simulink model "SbWModel"  (R2018a)
settings: Solver=FixedStepDiscrete  StartTime=0.0  StopTime=inf  FixedStep=0.002  RelTol=1e-3  EnableMultiTasking=on
values from neighbouring files (symbols this model uses):
  Bsc = 0.136    [SBWData.m]
  Im1 = 0.0021    [SBWData.m]
  Isw = 0.0079    [SBWData.m]
  Kb1 = 0.35    [SBWData.m]
  Ks1 = 3500    [SBWData.m]
  m = 1573    [STData.m]
  R1 = 4.6    [SBWData.m]
  RR = m*Csf    (= 34.606)    [STData.m]
  Tsmall = 0.001    [STData.m]
undefined symbols (not defined in the file or in its folder): Bm1, kt1, Tfr_c
settings Model: ExtModeTrigDuration=10000  Creator=srivats  LastModifiedBy=srivats
settings SolverCC: PositivePriorityOrder=on
settings RTWCC: SystemTargetFile=quarc_win64.tlc  TemplateMakefile=quarc_default_tmf  Description=QUARC Win64 Target
settings STFCustomTargetCC: TargetPreCompLibLocation=C:\PROGRA~3\QUARC\lib\2018a\win64\release  TargetLangStandard=C99 (ISO)  ConcurrentExecutionCompliant=on  SystemTargetFile=quarc_win64.tlc
settings GRTTargetCC: TargetPreCompLibLocation=C:\PROGRA~3\QUARC\lib\2018a\win64\release  ParMdlRefBuildCompliant=off  CompOptLevelCompliant=off  CombineOutputUpdateFcns=off  MatFileLogging=off  CPPClassGenCompliant=off  GRTInterface=on  UseToolchainInfoCompliant=off  ExtMode=on  ExtModeMexFile=quarc_comm

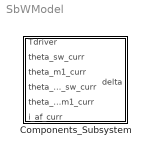
== system SbWModel ==
  Components_Subsystem : Subsystem

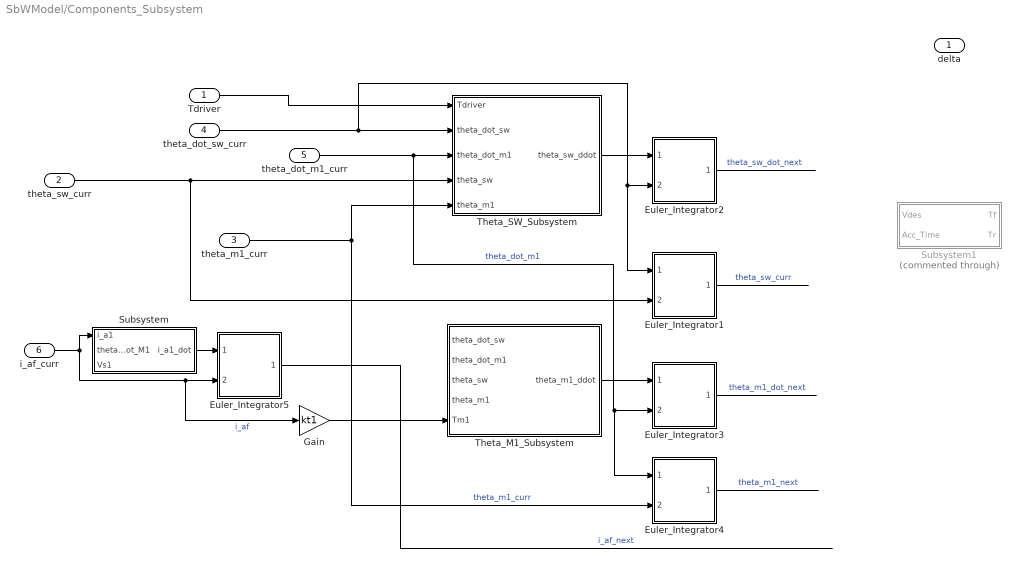
== system SbWModel/Components_Subsystem ==
  Tdriver : Inport
  theta_sw_curr : Inport  Port=2
  theta_m1_curr : Inport  Port=3
  theta_dot_sw_curr : Inport  Port=4
  theta_dot_m1_curr : Inport  Port=5
  i_af_curr : Inport  Port=6
  Euler_Integrator1 : Subsystem
  Euler_Integrator2 : Subsystem
  Euler_Integrator3 : Subsystem
  Euler_Integrator4 : Subsystem
  Euler_Integrator5 : Subsystem
  Gain : Gain  Gain=kt1
  Subsystem : Subsystem
  Subsystem1 : Subsystem  Commented=through
  Theta_M1_Subsystem : Subsystem
  Theta_SW_Subsystem : Subsystem
  delta : Outport
  wires:
  Tdriver/1 -> Theta_SW_Subsystem/1(Tdriver)
  theta_dot_sw_curr/1 -> Euler_Integrator1/1(state_dot), Euler_Integrator2/2(state_curr), Theta_SW_Subsystem/2(theta_dot_sw)
  theta_dot_m1_curr/1 -> Euler_Integrator4/1(state_dot), Euler_Integrator3/2(state_curr), Theta_SW_Subsystem/3(theta_dot_m1)  "theta_dot_m1"
  theta_sw_curr/1 -> Euler_Integrator1/2(state_curr), Theta_SW_Subsystem/4(theta_sw)
  theta_m1_curr/1 -> Euler_Integrator4/2(state_curr), Theta_SW_Subsystem/5(theta_m1)  "theta_m1_curr"
  Theta_SW_Subsystem/1(theta_sw_ddot) -> Euler_Integrator2/1(state_dot)
  Euler_Integrator2/1(state_next) -> ?  "theta_sw_dot_next"
  Euler_Integrator1/1(state_next) -> ?  "theta_sw_curr"
  Theta_M1_Subsystem/1("theta_m1_ddot ") -> Euler_Integrator3/1(state_dot)
  Euler_Integrator3/1(state_next) -> ?  "theta_m1_dot_next"
  Euler_Integrator4/1(state_next) -> ?  "theta_m1_next"
  i_af_curr/1 -> Gain/1, Euler_Integrator5/2(state_curr), Subsystem/1(i_a1)  "i_af"
  Subsystem/1(i_a1_dot) -> Euler_Integrator5/1(state_dot)
  Euler_Integrator5/1(state_next) -> ?  "i_af_next"
  Gain/1 -> Theta_M1_Subsystem/5(Tm1)

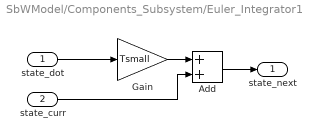
== system SbWModel/Components_Subsystem/Euler_Integrator1 ==
  state_dot : Inport
  state_curr : Inport  Port=2
  Add : Sum
  Gain : Gain  Gain=Tsmall
  state_next : Outport
  wires:
  state_dot/1 -> Gain/1
  Gain/1 -> Add/1
  state_curr/1 -> Add/2
  Add/1 -> state_next/1

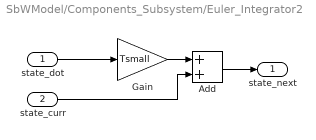
== system SbWModel/Components_Subsystem/Euler_Integrator2 ==
  state_dot : Inport
  state_curr : Inport  Port=2
  Add : Sum
  Gain : Gain  Gain=Tsmall
  state_next : Outport
  wires:
  state_dot/1 -> Gain/1
  Gain/1 -> Add/1
  state_curr/1 -> Add/2
  Add/1 -> state_next/1

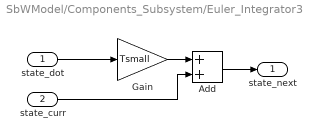
== system SbWModel/Components_Subsystem/Euler_Integrator3 ==
  state_dot : Inport
  state_curr : Inport  Port=2
  Add : Sum
  Gain : Gain  Gain=Tsmall
  state_next : Outport
  wires:
  state_dot/1 -> Gain/1
  Gain/1 -> Add/1
  state_curr/1 -> Add/2
  Add/1 -> state_next/1

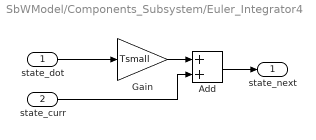
== system SbWModel/Components_Subsystem/Euler_Integrator4 ==
  state_dot : Inport
  state_curr : Inport  Port=2
  Add : Sum
  Gain : Gain  Gain=Tsmall
  state_next : Outport
  wires:
  state_dot/1 -> Gain/1
  Gain/1 -> Add/1
  state_curr/1 -> Add/2
  Add/1 -> state_next/1

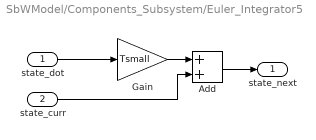
== system SbWModel/Components_Subsystem/Euler_Integrator5 ==
  state_dot : Inport
  state_curr : Inport  Port=2
  Add : Sum
  Gain : Gain  Gain=Tsmall
  state_next : Outport
  wires:
  state_dot/1 -> Gain/1
  Gain/1 -> Add/1
  state_curr/1 -> Add/2
  Add/1 -> state_next/1

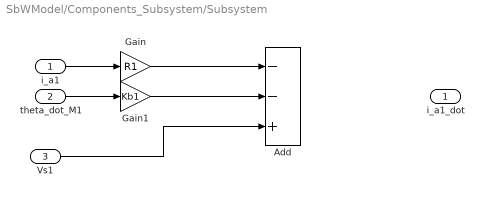
== system SbWModel/Components_Subsystem/Subsystem ==
  i_a1 : Inport
  theta_dot_M1 : Inport  Port=2
  Vs1 : Inport  Port=3
  Add : Sum  Inputs=--+
  Gain : Gain  Gain=R1
  Gain1 : Gain  Gain=Kb1
  i_a1_dot : Outport
  wires:
  Gain/1 -> Add/1
  Gain1/1 -> Add/2
  i_a1/1 -> Gain/1
  theta_dot_M1/1 -> Gain1/1
  Vs1/1 -> Add/3

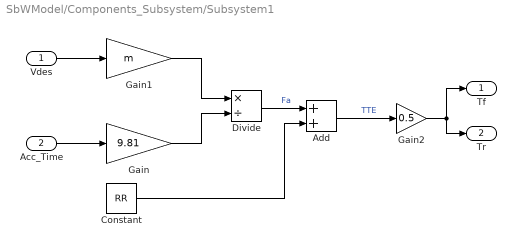
== system SbWModel/Components_Subsystem/Subsystem1 ==
  Vdes : Inport
  Acc_Time : Inport  Port=2
  Add : Sum
  Constant : Constant  Value=RR
  Divide : Product  Inputs=*/
  Gain : Gain  Gain=9.81
  Gain1 : Gain  Gain=m
  Gain2 : Gain  Gain=0.5
  Tf : Outport
  Tr : Outport  Port=2
  wires:
  Vdes/1 -> Gain1/1
  Acc_Time/1 -> Gain/1
  Gain1/1 -> Divide/1
  Gain/1 -> Divide/2
  Divide/1 -> Add/1  "Fa"
  Constant/1 -> Add/2
  Add/1 -> Gain2/1  "TTE"
  Gain2/1 -> Tf/1, Tr/1

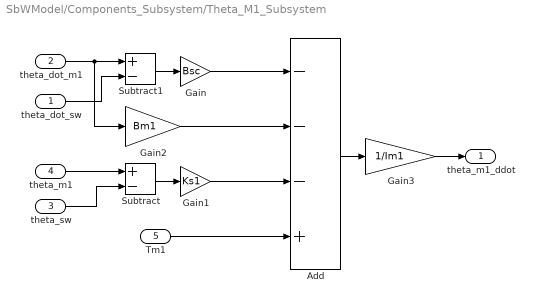
== system SbWModel/Components_Subsystem/Theta_M1_Subsystem ==
  theta_dot_sw : Inport
  theta_dot_m1 : Inport  Port=2
  theta_sw : Inport  Port=3
  theta_m1 : Inport  Port=4
  Tm1 : Inport  Port=5
  Add : Sum  Inputs=---+
  Gain : Gain  Gain=Bsc
  Gain1 : Gain  Gain=Ks1
  Gain2 : Gain  Gain=Bm1
  Gain3 : Gain  Gain=1/Im1
  Subtract : Sum  Inputs=+-
  Subtract1 : Sum  Inputs=+-
  "theta_m1_ddot " : Outport
  wires:
  theta_m1/1 -> Subtract/1
  theta_sw/1 -> Subtract/2
  theta_dot_m1/1 -> Gain2/1, Subtract1/1
  theta_dot_sw/1 -> Subtract1/2
  Subtract/1 -> Gain1/1
  Subtract1/1 -> Gain/1
  Gain/1 -> Add/1
  Gain1/1 -> Add/3
  Gain2/1 -> Add/2
  Tm1/1 -> Add/4
  Add/1 -> Gain3/1
  Gain3/1 -> "theta_m1_ddot "/1

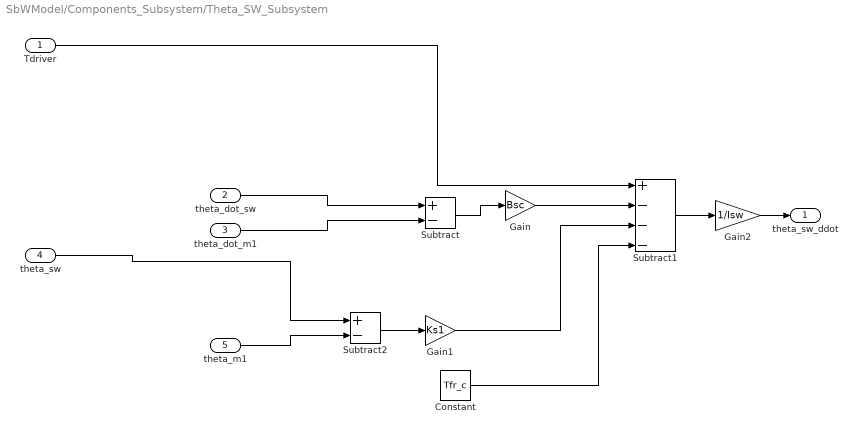
== system SbWModel/Components_Subsystem/Theta_SW_Subsystem ==
  Tdriver : Inport
  theta_dot_sw : Inport  Port=2
  theta_dot_m1 : Inport  Port=3
  theta_sw : Inport  Port=4
  theta_m1 : Inport  Port=5
  Constant : Constant  Value=Tfr_c
  Gain : Gain  Gain=Bsc
  Gain1 : Gain  Gain=Ks1
  Gain2 : Gain  Gain=1/Isw
  Subtract : Sum  Inputs=+-
  Subtract1 : Sum  Inputs=+---
  Subtract2 : Sum  Inputs=+-
  theta_sw_ddot : Outport
  wires:
  Subtract/1 -> Gain/1
  Constant/1 -> Subtract1/4
  theta_m1/1 -> Subtract2/2
  theta_sw/1 -> Subtract2/1
  Gain/1 -> Subtract1/2
  theta_dot_m1/1 -> Subtract/2
  theta_dot_sw/1 -> Subtract/1
  Subtract1/1 -> Gain2/1
  Gain1/1 -> Subtract1/3
  Subtract2/1 -> Gain1/1
  Tdriver/1 -> Subtract1/1
  Gain2/1 -> theta_sw_ddot/1
